simulink model "progetto3NO_LQG"  (Simulink 7.9)
settings: Solver=ode23s  StartTime=0.0  StopTime=80  RelTol=1e-3
values from neighbouring files (symbols this model uses):
  AMI = AK1    [AstaDecoupleV2.m]    (also in AstaDecoupleV3.m; AstaTenzoV2.m; AstaTenzoV3.m)
  AMin = [ ... (first row only)    [AstaDecoupleV2.m]    (also in AstaDecoupleV3.m; AstaTenzoV2.m; AstaTenzoV3.m)
  Aoss = AMin-V*ClocalMin    [AstaDecoupleV2.m]    (also in AstaDecoupleV3.m; AstaTenzoV2.m; AstaTenzoV3.m)
  BMI = BK1    [AstaDecoupleV2.m]    (also in AstaDecoupleV3.m; AstaTenzoV2.m; AstaTenzoV3.m)
  Bmod = [M BMin]    [AstaDecoupleV2.m]    (also in AstaDecoupleV3.m; AstaTenzoV2.m; AstaTenzoV3.m)
  Boss = [BMin-V*D V M-V*N]    [AstaDecoupleV2.m]    (also in AstaDecoupleV3.m; AstaTenzoV2.m; AstaTenzoV3.m)
  ClocalMin = [ ... (first row only)    [AstaDecoupleV2.m]    (also in AstaDecoupleV3.m; AstaTenzoV2.m; AstaTenzoV3.m)
  CMI = eye(q*mu)    [AstaDecoupleV2.m]    (also in AstaDecoupleV3.m; AstaTenzoV2.m; AstaTenzoV3.m)
  Coss = eye(n)    [AstaDecoupleV2.m]    (also in AstaDecoupleV3.m; AstaTenzoV2.m; AstaTenzoV3.m)
  D_phi = [1 325.437715018286 23852.1596168943 0]    [AstaDecoupleV2.m]    (also in AstaDecoupleV3.m; AstaTenzoV3.m)
  D_psi = [1 378.139322580724 35127.9961825618 0]    [AstaDecoupleV2.m]    (also in AstaDecoupleV3.m = [1 325.437715018286 23852.1596168943 0]; AstaTenzoV3.m)
  D_theta = [1 325.437715018286 23852.1596168943 0]    [AstaDecoupleV2.m]    (also in AstaDecoupleV3.m; AstaTenzoV3.m)
  D_thrust = [1 963.786798861645 190423.384445206 0]    [AstaDecoupleV2.m]    (also in AstaDecoupleV3.m = [1 888.737639530835 157281.746006557]; AstaTenzoV3.m)
  DMI = zeros(q*mu,q)    [AstaDecoupleV2.m]    (also in AstaDecoupleV3.m; AstaTenzoV2.m; AstaTenzoV3.m)
  Dmod = [N D]    [AstaDecoupleV2.m]    (also in AstaDecoupleV3.m; AstaTenzoV2.m; AstaTenzoV3.m)
  Doss = zeros(size(Boss))    [AstaDecoupleV2.m]    (also in AstaDecoupleV3.m; AstaTenzoV2.m; AstaTenzoV3.m)
  F1 = F(:,size(AMin,1)+1:size(F,2))    [AstaDecoupleV2.m]    (also in AstaDecoupleV3.m; AstaTenzoV2.m; AstaTenzoV3.m)
  F2 = F(:,1:size(AMin,1))    [AstaDecoupleV2.m]    (also in AstaDecoupleV3.m; AstaTenzoV2.m; AstaTenzoV3.m)
  N_phi = [440.513056398418 26779.6272064186          272303.182447317 584729.91630594]    [AstaDecoupleV2.m]    (also in AstaDecoupleV3.m; AstaTenzoV3.m)
  N_psi = [59260.0621820611 3429565.45270113           27702908.9364068 53625940.9126871]    [AstaDecoupleV2.m]    (also in AstaDecoupleV3.m = [440.513056398418 26779.6272064186          272303.182447317; AstaTenzoV3.m)
  N_theta = [440.513056398418 26779.6272064186          272303.182447317 584729.91630594]    [AstaDecoupleV2.m]    (also in AstaDecoupleV3.m; AstaTenzoV3.m)
  N_thrust = [682900.887332905 4668183.15145263]    [AstaDecoupleV2.m]    (also in AstaDecoupleV3.m = [2882048.25903061 3827833.12977005]; AstaTenzoV3.m)
  omega = 0.5    [AstaDecoupleV2.m]    (also in AstaDecoupleV3.m; AstaTenzoV2.m; AstaTenzoV3.m)
libraries: simulink x1
settings Model: Creator=danilo  LastModifiedBy=userk
settings DebuggingCC: FcnCallInpInsideContextMsg=Use local settings
settings GRTTargetCC: CombineOutputUpdateFcns=off  GRTInterface=on

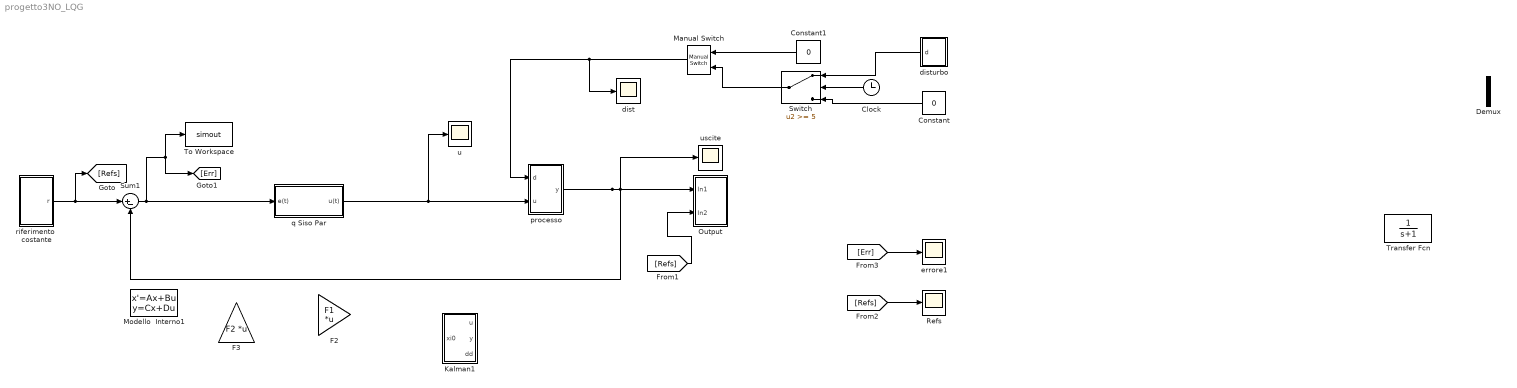
== system progetto3NO_LQG ==
  Clock : Clock
  Constant : Constant  Value=0
  Constant1 : Constant  Value=0
  Demux : Demux  Outputs=2
  F2 : Gain  Gain=F1  Multiplication=Matrix(K*u) (u vector)
  F3 : Gain  Gain=F2  Multiplication=Matrix(K*u) (u vector)
  Kalman1 : Subsystem
  Manual Switch : simulink/Signal Routing/Manual Switch  sw=0  action=0  varsize=off
  Modello  Interno1 : StateSpace  A=AMI  B=BMI  C=CMI  D=DMI
  Output : Subsystem
  Refs : Scope
  Sum1 : Sum  Inputs=|+-
  Switch : Switch  Threshold=5
  To Workspace : ToWorkspace  VariableName=simout  SampleTime=-1  SaveFormat=Structure
  Transfer Fcn : TransferFcn  Denominator=[1 1]
  dist : Scope
      settings: SaveName=ScopeData5
  disturbo : Subsystem
  errore1 : Scope
      settings: SaveName=ScopeData8
  processo : Subsystem
  "q Siso Par " : Subsystem
  riferimento  costante : Subsystem
  u : Scope
      settings: SaveName=ScopeData3
  uscite : Scope
      settings: TimeRange=80  YMin=-17.45927637246444  YMax=15.6384603336206  SaveName=ScopeData2
  wires:
  riferimento  costante/1(r) -> Sum1/1, [Refs]
  processo/1(y) -> Sum1/2, Output/1(In1), uscite/1
  Sum1/1 -> To Workspace/1, [Err], "q Siso Par "/1(e(t))
  [Refs] -> Output/2(In2)
  [Refs] -> Refs/1
  [Err] -> errore1/1
  Clock/1 -> Switch/2
  disturbo/1(d) -> Switch/1
  Constant/1 -> Switch/3
  "q Siso Par "/1(u(t)) -> processo/2(u), u/1
  Constant1/1 -> Manual Switch/1
  Switch/1 -> Manual Switch/2
  Manual Switch/1 -> processo/1(d), dist/1

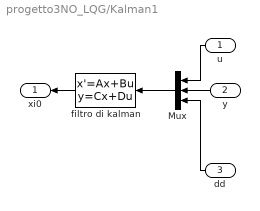
== system progetto3NO_LQG/Kalman1 ==
  u : Inport
  y : Inport  Port=2
  dd : Inport  Port=3
  Mux : Mux  Inputs=[4 4 1]
  filtro di kalman : StateSpace  A=Aoss  B=Boss  C=Coss  D=Doss
  xi0 : Outport
  wires:
  dd/1 -> Mux/3
  y/1 -> Mux/2
  filtro di kalman/1 -> xi0/1
  u/1 -> Mux/1
  Mux/1 -> filtro di kalman/1

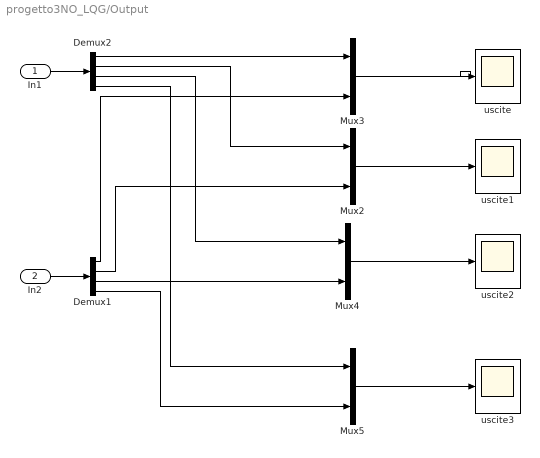
== system progetto3NO_LQG/Output ==
  In1 : Inport
  In2 : Inport  Port=2
  Demux1 : Demux
  Demux2 : Demux
  Mux{2..5} (4 alike) : Mux  Inputs=2
  uscite{,1..3} (4 alike) : Scope
      uscite settings: TickLabels=on  YMin=-3.5  YMax=7
      uscite1 settings: TickLabels=on  TimeRange=30  YMin=0.75  YMax=4.25  SaveName=ScopeData4
      uscite2 settings: TickLabels=on  YMin=0.75  YMax=4.25  SaveName=ScopeData6
      uscite3 settings: TickLabels=on  YMin=0.75  YMax=4.25  SaveName=ScopeData7
  wires:
  Demux1/1 -> Mux3/2
  In2/1 -> Demux1/1
  In1/1 -> Demux2/1
  Mux3/1 -> uscite/1
  Demux2/1 -> Mux3/1
  Mux2/1 -> uscite1/1
  Demux2/2 -> Mux2/1
  Mux4/1 -> uscite2/1
  Demux2/3 -> Mux4/1
  Mux5/1 -> uscite3/1
  Demux2/4 -> Mux5/1
  Demux1/2 -> Mux2/2
  Demux1/3 -> Mux4/2
  Demux1/4 -> Mux5/2

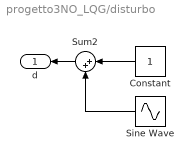
== system progetto3NO_LQG/disturbo ==
  Constant : Constant
  Sine Wave : Sin  Amplitude=3  Frequency=omega  SampleTime=0
  Sum2 : Sum  Inputs=|++
  d : Outport
  wires:
  Sine Wave/1 -> Sum2/2
  Constant/1 -> Sum2/1
  Sum2/1 -> d/1

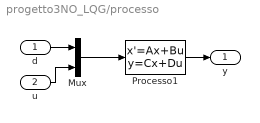
== system progetto3NO_LQG/processo ==
  d : Inport
  u : Inport  Port=2
  Mux : Mux  Inputs=[1 4]
  Processo1 : StateSpace  A=AMin  B=Bmod  C=ClocalMin  D=Dmod
  y : Outport
  wires:
  Mux/1 -> Processo1/1
  d/1 -> Mux/1
  Processo1/1 -> y/1
  u/1 -> Mux/2

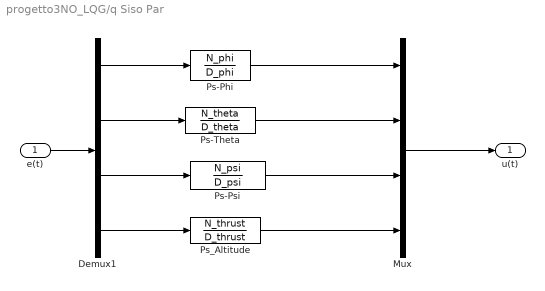
== system progetto3NO_LQG/q Siso Par  ==
  e(t) : Inport
  Demux1 : Demux
  Mux : Mux
  Ps-Phi : TransferFcn  Numerator=N_phi  Denominator=D_phi
  Ps-Psi : TransferFcn  Numerator=N_psi  Denominator=D_psi
  Ps-Theta : TransferFcn  Numerator=N_theta  Denominator=D_theta
  Ps_Altitude : TransferFcn  Numerator=N_thrust  Denominator=D_thrust
  u(t) : Outport
  wires:
  Mux/1 -> u(t)/1
  e(t)/1 -> Demux1/1
  Ps-Psi/1 -> Mux/3
  Ps-Theta/1 -> Mux/2
  Demux1/2 -> Ps-Theta/1
  Ps_Altitude/1 -> Mux/4
  Ps-Phi/1 -> Mux/1
  Demux1/4 -> Ps_Altitude/1
  Demux1/3 -> Ps-Psi/1
  Demux1/1 -> Ps-Phi/1

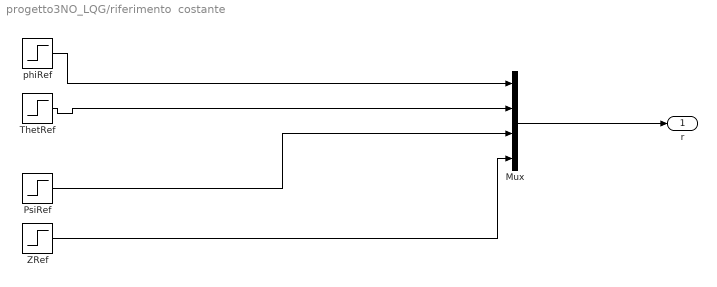
== system progetto3NO_LQG/riferimento  costante ==
  Mux : Mux  Inputs=[1 1 1 1]
  PsiRef : Step  Time=0.8  After=2.5  SampleTime=0
  ThetRef : Step  Time=0.5  After=2  SampleTime=0
  ZRef : Step  Time=3  After=2.5  SampleTime=0
  phiRef : Step  After=1.5  SampleTime=0
  r : Outport
  wires:
  Mux/1 -> r/1
  phiRef/1 -> Mux/1
  ThetRef/1 -> Mux/2
  PsiRef/1 -> Mux/3
  ZRef/1 -> Mux/4
